simulink model "mRobotArmControl"  (R2021a)
settings: Solver=FixedStepAuto  StartTime=0.0  StopTime=inf  RelTol=1e-3  EnableMultiTasking=on
InitFcn:
  | cBase=90;
  | cShoulder=90;
  | cElbow=90;
  | cWristVer=90;
  | cWristRot=90;
  | cGripper=73;
libraries: arduinolib x13
settings Model: SILPILModeSetting=veronly  ExtModeTrigDuration=2  Creator=loris  LastModifiedBy=angelo
settings OptimizationCC: EnhancedBackFolding=on  PassReuseOutputArgsAs=Individual arguments  ZeroExternalMemoryAtStartup=off  ZeroInternalMemoryAtStartup=off  MaxStackSize=64  OptimizeBlockOrder=speed  DifferentSizesBufferReuse=on  OptimizationCustomize=off  EfficientTunableParamExpr=on
settings DebuggingCC: ParameterTunabilityLossMsg=error
settings HardwareCC: ProdBitPerInt=16  ProdBitPerPointer=16  ProdBitPerSizeT=16  ProdBitPerPtrDiffT=16  ProdLargestAtomicFloat=None  ProdWordSize=8  ProdHWDeviceType=Atmel->AVR
settings SFSimCC: MATLABDynamicMemAlloc=off
settings RTWCC: SystemTargetFile=ert.tlc  HardwareBoard=Arduino Mega 2560  TemplateMakefile=ert_default_tmf  Toolchain=Arduino AVR  BuildConfiguration=Faster Runs
settings CodeAppCC: ForceParamTrailComments=on  IgnoreCustomStorageClasses=off  OperatorAnnotations=on  SimulinkDataObjDesc=on  SFDataObjDesc=on  InsertBlockDesc=on
settings ERTTargetCC: TargetLangStandard=C99 (ISO)  SupportContinuousTime=on  SupportVariableSizeSignals=on  ExtModeStaticAllocSize=2048  RootIOFormat=Structure reference

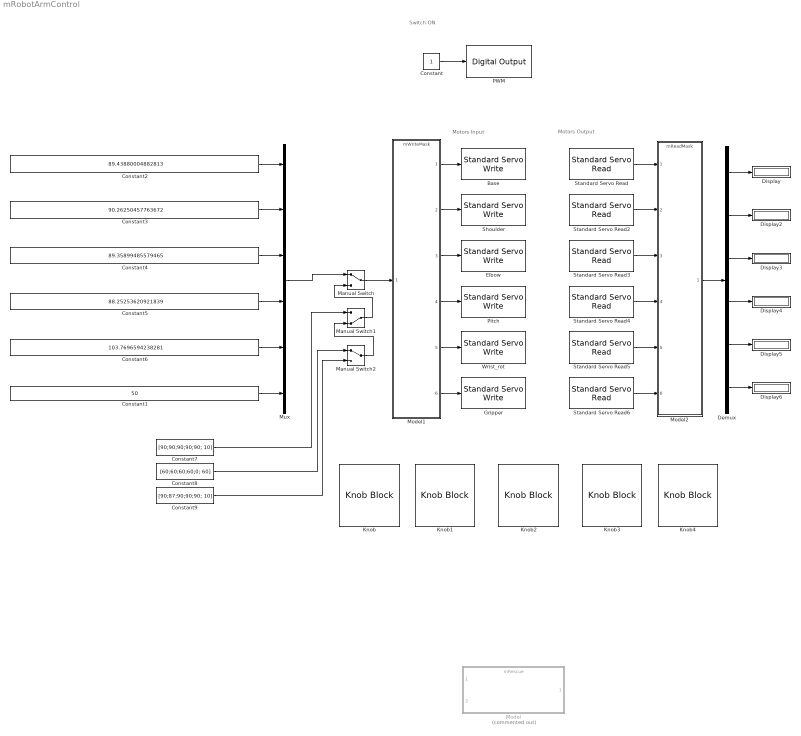
== system mRobotArmControl ==
  note: Motors Output
  note: Switch ON
  note: Motors Input
  Base : arduinolib/Standard Servo Write  pinNumber=11  ServoIndex=0  blockPlatform=ARDUINO
  Constant : Constant
  Constant1 : Constant  Value=50
  Constant2 : Constant  Value=89.43880004882813
  Constant3 : Constant  Value=90.26250457763672
  Constant4 : Constant  Value=89.35899485579465
  Constant5 : Constant  Value=88.25253620921839
  Constant6 : Constant  Value=103.7696594238281
  Constant7 : Constant  Value=[90;90;90;90;90; 10]
  Constant8 : Constant  Value=[60;60;60;60;0; 60]
  Constant9 : Constant  Value=[90;87;90;90;90; 10]
  Demux : Demux  Outputs=6
  Display{,2..6} (6 alike) : Display
  Elbow : arduinolib/Standard Servo Write  pinNumber=9  ServoIndex=1  blockPlatform=ARDUINO
  Gripper : arduinolib/Standard Servo Write  pinNumber=3  ServoIndex=2  blockPlatform=ARDUINO
  Knob{,2..4} (4 alike) : KnobBlock  ScaleMax=180
  Knob1 : KnobBlock  ScaleMin=15  ScaleMax=165
  Manual Switch : ManualSwitch
  Manual Switch1 : ManualSwitch  CurrentSetting=0
  Manual Switch2 : ManualSwitch
  Model : ModelReference  Commented=on  ModelNameDialog=mRescue.slx  SimulationMode=Normal  ModelReferenceVersion=1.5
  Model1 : ModelReference  ModelNameDialog=mWriteMask.slx  SimulationMode=Normal  ModelReferenceVersion=1.1
  Model2 : ModelReference  ModelNameDialog=mReadMask.slx  SimulationMode=Normal  ModelReferenceVersion=1.1
  Mux : Mux  Inputs=6
  PWM : arduinolib/Digital Output  pinNumber=12  Direction=output  blockPlatform=arduino
  Pitch : arduinolib/Standard Servo Write  pinNumber=6  ServoIndex=3  blockPlatform=ARDUINO
  Shoulder : arduinolib/Standard Servo Write  pinNumber=10  ServoIndex=4  blockPlatform=ARDUINO
  Standard Servo Read : arduinolib/Standard Servo Read  pinNumber=11  SampleTime=0.1  ServoIndex=0  blockPlatform=ARDUINO
      settings: SourceProductBaseCode=ARDUINO
  Standard Servo Read2 : arduinolib/Standard Servo Read  pinNumber=10  SampleTime=0.1  ServoIndex=4  blockPlatform=ARDUINO
      settings: SourceProductBaseCode=ARDUINO
  Standard Servo Read3 : arduinolib/Standard Servo Read  pinNumber=9  SampleTime=0.1  ServoIndex=1  blockPlatform=ARDUINO
      settings: SourceProductBaseCode=ARDUINO
  Standard Servo Read4 : arduinolib/Standard Servo Read  pinNumber=6  SampleTime=0.1  ServoIndex=3  blockPlatform=ARDUINO
      settings: SourceProductBaseCode=ARDUINO
  Standard Servo Read5 : arduinolib/Standard Servo Read  pinNumber=5  SampleTime=0.1  ServoIndex=5  blockPlatform=ARDUINO
      settings: SourceProductBaseCode=ARDUINO
  Standard Servo Read6 : arduinolib/Standard Servo Read  pinNumber=3  SampleTime=0.1  ServoIndex=2  blockPlatform=ARDUINO
      settings: SourceProductBaseCode=ARDUINO
  Wrist_rot : arduinolib/Standard Servo Write  pinNumber=5  ServoIndex=5  blockPlatform=ARDUINO
  wires:
  Constant/1 -> PWM/1
  Constant4/1 -> Mux/3
  Constant5/1 -> Mux/4
  Constant6/1 -> Mux/5
  Constant1/1 -> Mux/6
  Constant3/1 -> Mux/2
  Constant2/1 -> Mux/1
  Mux/1 -> Manual Switch/1
  Demux/1 -> Display/1
  Demux/2 -> Display2/1
  Demux/3 -> Display3/1
  Demux/4 -> Display4/1
  Demux/5 -> Display5/1
  Demux/6 -> Display6/1
  Constant7/1 -> Manual Switch1/1
  Manual Switch1/1 -> Manual Switch/2
  Constant8/1 -> Manual Switch2/1
  Constant9/1 -> Manual Switch2/2
  Manual Switch2/1 -> Manual Switch1/2
  Manual Switch/1 -> Model1/1
  Model1/1 -> Base/1
  Model1/2 -> Shoulder/1
  Model1/3 -> Elbow/1
  Model1/4 -> Pitch/1
  Model1/5 -> Wrist_rot/1
  Model1/6 -> Gripper/1
  Standard Servo Read/1 -> Model2/1
  Standard Servo Read2/1 -> Model2/2
  Standard Servo Read3/1 -> Model2/3
  Standard Servo Read4/1 -> Model2/4
  Standard Servo Read5/1 -> Model2/5
  Standard Servo Read6/1 -> Model2/6
  Model2/1 -> Demux/1
